simulink model "test_drone"  (R2023b)
settings: Solver=VariableStepAuto  StartTime=0.0  StopTime=10.0  RelTol=1e-3
undefined symbols (not defined in the file or in its folder): t_sample, x_init, y_init, z_init
libraries: uavsim3dlib x1, sim3dphyssensorlib x1, simulink x1
settings Model: Creator=matte  LastModifiedBy=matte

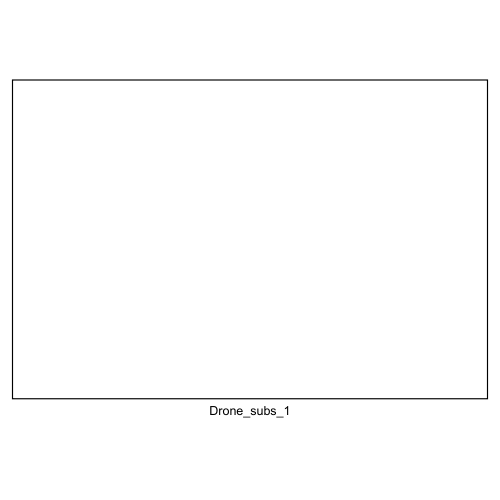
[thumbnail: Simulink's stored preview of the top-level diagram]
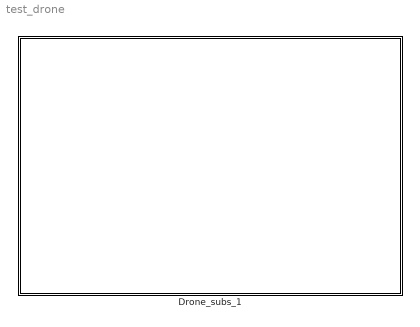
== system test_drone ==
  Drone_subs_1 : Subsystem

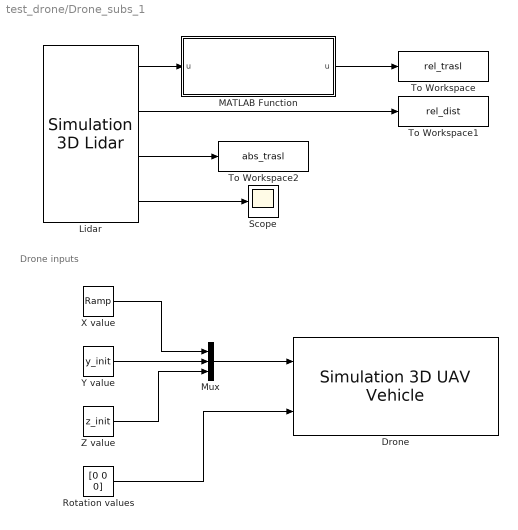
== system test_drone/Drone_subs_1 ==
  note: Drone inputs
  Drone : uavsim3dlib/Simulation 3D UAV Vehicle  Priority=-1  Mesh=Quadrotor  MeshPath=/MathWorksUAVContent/UAVs/HexaRotorUAV/HexaRotor.HexaRotor  Color=Black  ActorName=SimulinkVehicle1  UseGlobalFrame=off  InitialTranslation=[x_init y_init z_init]  InitialRotation=[0 0 0]  InitialTranslationGlobal=[0 0 0]  InitialGeoOrigin=[0 0 0]  InitialRotationGlobal=[0 0 0]  SampleTime=-1  ActorType=SimulinkVehicle  ID=1  aMode=4  ActorTag=SimulinkVehicle1
  Lidar : sim3dphyssensorlib/Simulation 3D Lidar  Priority=-1  sensorTag=Sim3dSensor1  sensorId=1  sensorName=Sim3dSensor1  vehTagList={'Scene Origin';'SimulinkVehicle1'}  vehTag=SimulinkVehicle1  mountLoc=Origin  offsetFlag=on  tmountOffset=[0, 0, -0.2]  rmountOffset=[0, 0, 0]  DetectionRange=50  RangeResolution=0.1  VerticalFOV=0.1  VerticalResolution=0.1  HorizontalFOV=360  HorizontalResolution=1  DistanceOutportEnabled=on  ReflectivityOutportEnabled=off  SemanticOutportEnabled=off  TransformOutportEnabled=on  SampleTime=t_sample  mountPoint=[0 0 -0.2]  mountOrientation=[0 0 0]  aMode=4  ID=1
      settings: LibrarySourceBlock=uavsim3dlib/Simulation 3D Lidar
  MATLAB Function : MATLAB Function  TreatAsAtomicUnit=on
  Mux : Mux  Inputs=3
  Rotation values : Constant  Value=[0 0 0]
  Scope : Scope
  To Workspace : ToWorkspace  VariableName=rel_trasl  SaveFormat=Structure  SampleTime=-1
      settings: Save2DSignal=2-D array (concatenate along first dimension)
  To Workspace1 : ToWorkspace  VariableName=rel_dist  SaveFormat=Structure  SampleTime=-1
      settings: Save2DSignal=2-D array (concatenate along first dimension)
  To Workspace2 : ToWorkspace  VariableName=abs_trasl  SaveFormat=Structure  SampleTime=-1
      settings: Save2DSignal=2-D array (concatenate along first dimension)
  X value : simulink/Sources/Ramp  slope=5  start=0  InitialOutput=x_init
  Y value : Constant  Value=y_init
  Z value : Constant  Value=z_init
  wires:
  X value/1 -> Mux/1
  Lidar/3 -> To Workspace2/1
  Y value/1 -> Mux/2
  Lidar/4 -> Scope/1
  Lidar/2 -> To Workspace1/1
  Z value/1 -> Mux/3
  Mux/1 -> Drone/1
  Rotation values/1 -> Drone/2
  Lidar/1 -> MATLAB Function/1("u ")
  MATLAB Function/1(u) -> To Workspace/1

== matlab function test_drone/Drone_subs_1/MATLAB Function ==
  data: u input; u output
function u  = pointCloudVisualization(u)
    % u è l'input del blocco MATLAB Function, che rappresenta la matrice Point Cloud [1x2000x3]
    
    % Estrai le coordinate x, y, z dalla matrice di punti
    x = squeeze(u(1,:,1)); % Coordinate x
    y = squeeze(u(1,:,2)); % Coordinate y
    plot(y, x, '.');
    grid on;
    xlim([-50, 50]);
    ylim([-50, 50]);
    axis equal;

    % Aggiungi etichette degli assi e un titolo al grafico
    xlabel('X');
    ylabel('Y');
    title('Point Cloud Visualization');
end
